simulink model "modelGreenHydrogenPlant"  (R2025a)
settings: Solver=ode1  StartTime=0.0  StopTime=exe.tsim  FixedStep=exe.tstep  RelTol=1e-3
undefined symbols (not defined in the file): Chosen_Strategy, DiscIntNeverNeededParam, ELY, ESS, exe, fb, Grid, grid, Ib2, Kc, kd, Ki_cc_cp, Ki_Inertia_Less, Kp_cc_cp, kp_GFo, Kp_Inertia_Less, PV, R, Rload, Sb, SCLR, t_ELY_on, Theta_Vvsc0, Time_Step, Va0, Vb0, Vb1, Vb2, Vc0, Vm0, VSC01_id0, Vvsc0, wb, Zb
libraries: spsSeriesRLCBranchLib x18, spsCurrentMeasurementLib x17, spsVoltageMeasurementLib x15, Control_Lib x13, spsRMSLib x8, simulink x8, spsabctodq0Lib x7, spsThreePhaseBreakerLib x5, spsPowerdq0InstantaneousLib x4, spsGroundLib x3, spsUniversalBridgeLib x3, spsControlledVoltageSourceLib x3
(part 2 of 3)

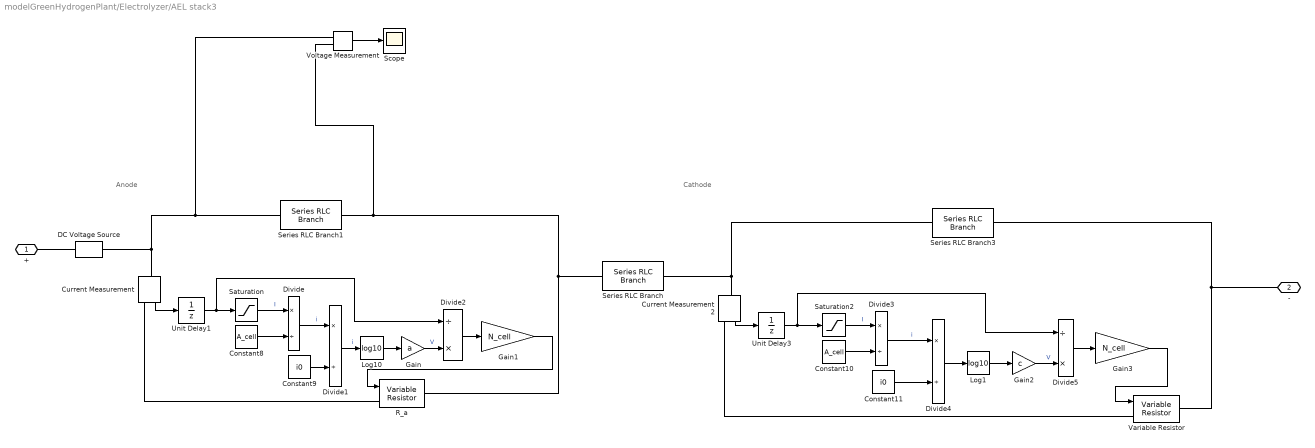
== system modelGreenHydrogenPlant/Electrolyzer/AEL stack3 ==
  note: Cathode
  note: Anode
  Constant10 : Constant  Value=A_cell
  Constant11 : Constant  Value=i0
  Constant8 : Constant  Value=A_cell
  Constant9 : Constant  Value=i0
  Current Measurement : spsCurrentMeasurementLib/Current Measurement  PhasorSimulation=off  OutputType=Complex  PSBequivalent=0
  Current Measurement2 : spsCurrentMeasurementLib/Current Measurement  PhasorSimulation=off  OutputType=Complex  PSBequivalent=0
  DC Voltage Source : spsDCVoltageSourceLib/DC Voltage Source  Amplitude=V_rev*N_cell  Measurements=None
  Divide{,1,3..4} (4 alike) : Product  Inputs=*/
  Divide2 : Product  Inputs=/*
  Divide5 : Product  Inputs=/*
  Gain : Gain  Gain=a
  Gain1 : Gain  Gain=N_cell
  Gain2 : Gain  Gain=c
  Gain3 : Gain  Gain=N_cell
  Log1 : Math  Operator=log10
  Log10 : Math  Operator=log10
  R_a : spsVariableResistorLib/Variable Resistor  Rabsmin=1e-3
      settings: LibrarySourceBlock=sps_lib/Passives/Variable Resistor
  Saturation : Saturate  UpperLimit=inf  LowerLimit=1e-3
  Saturation2 : Saturate  UpperLimit=inf  LowerLimit=1e-3
  Scope : Scope
      settings: ActiveDisplayYMinimum=40.73121  ActiveDisplayYMaximum=40.85796
  Series RLC Branch : spsSeriesRLCBranchLib/Series RLC Branch  LConnTagsString=__new0  RConnTagsString=__new0  BranchType=R  Resistance=R_cell_ohm/A_cell*N_cell  Inductance=1e-3  SetiL0=off  InitialCurrent=0  Capacitance=1e-6  Setx0=off  InitialVoltage=0  Measurements=None
  Series RLC Branch1 : spsSeriesRLCBranchLib/Series RLC Branch  LConnTagsString=__new0  RConnTagsString=__new0  BranchType=C  Resistance=1  Inductance=1e-3  SetiL0=off  InitialCurrent=0  Capacitance=Ca*A_cell *1e-3/N_cell  Setx0=on  InitialVoltage=V0_a_cell*N_cell  Measurements=None
  Series RLC Branch3 : spsSeriesRLCBranchLib/Series RLC Branch  LConnTagsString=__new0  RConnTagsString=__new0  BranchType=C  Resistance=1  Inductance=1e-3  SetiL0=off  InitialCurrent=0  Capacitance=Cc*A_cell *1e-3/N_cell  Setx0=on  InitialVoltage=V0_a_cell*N_cell  Measurements=None
  Unit Delay1 : UnitDelay  InitialCondition=I0_a  SampleTime=-1  HasFrameUpgradeWarning=on
  Unit Delay3 : UnitDelay  InitialCondition=I0_c  SampleTime=-1  HasFrameUpgradeWarning=on
  Variable Resistor : spsVariableResistorLib/Variable Resistor  Rabsmin=1e-3
      settings: LibrarySourceBlock=sps_lib/Passives/Variable Resistor
  Voltage Measurement : spsVoltageMeasurementLib/Voltage Measurement  PhasorSimulation=off  OutputType=Complex  PSBequivalent=0
  + : PMIOPort  Side=Left
  - : PMIOPort  Port=2  Side=Right
  wires:
  Saturation/1 -> Divide/1  "I"
  Constant8/1 -> Divide/2
  Gain/1 -> Divide2/2  "V"
  Gain1/1 -> R_a/1
  Divide2/1 -> Gain1/1
  Log10/1 -> Gain/1
  Current Measurement/1 -> Unit Delay1/1
  Current Measurement2/1 -> Unit Delay3/1
  Saturation2/1 -> Divide3/1  "I"
  Gain3/1 -> Variable Resistor/1
  Constant10/1 -> Divide3/2
  Divide5/1 -> Gain3/1
  Gain2/1 -> Divide5/2  "V"
  Divide4/1 -> Log1/1
  Log1/1 -> Gain2/1
  Constant11/1 -> Divide4/2
  Divide3/1 -> Divide4/1  "i"
  Divide/1 -> Divide1/1  "i"
  Constant9/1 -> Divide1/2
  Divide1/1 -> Log10/1  "i"
  Unit Delay1/1 -> Saturation/1, Divide2/1
  Unit Delay3/1 -> Divide5/1, Saturation2/1
  Voltage Measurement/1 -> Scope/1
  connections:
  R_a/RConn1 -- Voltage Measurement/LConn2 -- Series RLC Branch1/RConn1 -- Series RLC Branch/LConn1
  +/RConn1 -- DC Voltage Source/RConn1
  Current Measurement/RConn1 -- R_a/LConn1
  Series RLC Branch/RConn1 -- Current Measurement2/LConn1 -- Series RLC Branch3/LConn1
  Current Measurement2/RConn1 -- Variable Resistor/LConn1
  -/RConn1 -- Variable Resistor/RConn1 -- Series RLC Branch3/RConn1
  DC Voltage Source/LConn1 -- Current Measurement/LConn1 -- Voltage Measurement/LConn1 -- Series RLC Branch1/LConn1

== system modelGreenHydrogenPlant/Electrolyzer/Current Controller  ==
  Idref : Inport
  Iqref : Inport  Port=2
  Id : Inport  Port=3
  Iq : Inport  Port=4
  Vd : Inport  Port=5
  Vq : Inport  Port=6
  w : Inport  Port=7
  wt : Inport  Port=8
  Constant2 : Constant  Value=0
  Gain : Gain  Gain=ELY.CC.Kp
  Gain1 : Gain  Gain=ELY.CC.Ki
  Gain2 : Gain  Gain=ELY.CC.Kp
  Gain3 : Gain  Gain=ELY.CC.Ki
  Gain4 : Gain  Gain=ELY.CC.Lf
  Integrator : Integrator
  Integrator1 : Integrator
  Mux3 : Mux  Inputs=3
  Product : Product
  Product1 : Product
  Scope : Scope  NumInputPorts=2
      settings: ActiveDisplayYMinimum=-28.76857  ActiveDisplayYMaximum=18.72667
  Sum : Sum  Inputs=|+-
  Sum1 : Sum  Inputs=-+|
  Sum2 : Sum  Inputs=|++
  Sum3 : Sum  Inputs=|++
  Sum4 : Sum  Inputs=++-
  Sum5 : Sum  Inputs=+++
  dq0 to abc : spsdq0toabcLib/dq0 to abc  Alignment=90 degrees behind phase A axis
  Uref : Outport
  wires:
  Product/1 -> Sum4/3
  Product1/1 -> Sum5/1
  Idref/1 -> Sum/1
  Sum3/1 -> Sum5/2
  Integrator/1 -> Sum2/2
  Sum4/1 -> Mux3/1
  Integrator1/1 -> Sum3/2
  Constant2/1 -> Mux3/3
  Sum/1 -> Scope/1, Gain1/1, Gain/1
  Vd/1 -> Sum4/1
  Gain3/1 -> Integrator1/1
  Gain2/1 -> Sum3/1
  Gain/1 -> Sum2/1
  Gain4/1 -> Product/2, Product1/1
  Iq/1 -> Product/1, Sum1/1
  Id/1 -> Product1/2, Sum/2
  Sum2/1 -> Scope/2, Sum4/2
  Sum5/1 -> Mux3/2
  Sum1/1 -> Gain3/1, Gain2/1
  Gain1/1 -> Integrator/1
  Mux3/1 -> dq0 to abc/1
  dq0 to abc/1 -> Uref/1
  Iqref/1 -> Sum1/2
  w/1 -> Gain4/1
  wt/1 -> dq0 to abc/2
  Vq/1 -> Sum5/3

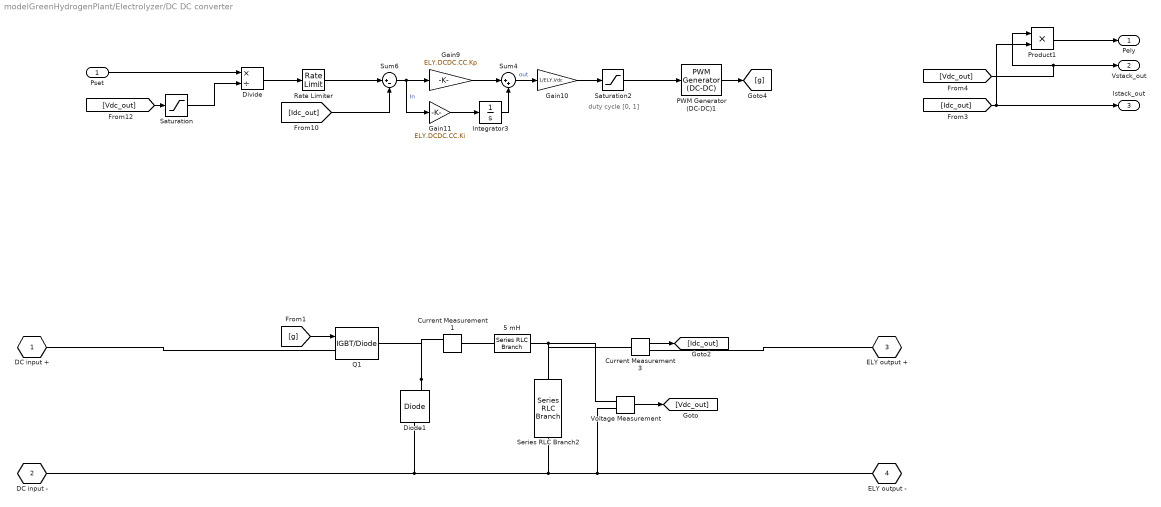
== system modelGreenHydrogenPlant/Electrolyzer/DC DC converter ==
  note: duty cycle [0, 1]
  Pset : Inport
  5 mH : spsSeriesRLCBranchLib/Series RLC Branch  LConnTagsString=__new0  RConnTagsString=__new0  BranchType=L  Resistance=ELY.DCDC.R_L  Inductance=ELY.DCDC.L  SetiL0=off  InitialCurrent=30  Capacitance=1.0  Setx0=off  InitialVoltage=0  Measurements=None
  Current Measurement1 : spsCurrentMeasurementLib/Current Measurement  PhasorSimulation=off  OutputType=Complex  PSBequivalent=0
  Current Measurement3 : spsCurrentMeasurementLib/Current Measurement  PhasorSimulation=off  OutputType=Complex  PSBequivalent=0
  Diode1 : spsDiodeLib/Diode  Ron=1e-3  Lon=0  Vf=0  IC=0  UseSnubber=off  Rs=inf  Cs=inf  Measurements=on
  Divide : Product  Inputs=*/
  Gain10 : Gain  Gain=1/ELY.Vdc
  Gain11 : Gain  Gain=ELY.DCDC.CC.Ki
  Gain9 : Gain  Gain=ELY.DCDC.CC.Kp
  Integrator3 : Integrator
  PWM Generator (DC-DC)1 : spsPWMGeneratorDCDCLib/PWM Generator (DC-DC)  Fsw=ELY.DCDC.fsw  Ts=0
  Product1 : Product
  Q1 : spsIGBTDiodeLib/IGBT//Diode  Ron=1e-3  Rs=1e5  Cs=inf  Measurements=off
  Rate Limiter : RateLimiter  RisingSlewLimit=ELY.DCDC.P.ramp.upperlimit  FallingSlewLimit=ELY.DCDC.P.ramp.lowerlimit  SampleTimeMode=inherited
  Saturation : Saturate  UpperLimit=inf  LowerLimit=95
  Saturation2 : Saturate  UpperLimit=1  LowerLimit=0
  Series RLC Branch2 : spsSeriesRLCBranchLib/Series RLC Branch  LConnTagsString=__new0  RConnTagsString=__new0  BranchType=C  Resistance=ELY.DCDC.R_C  Inductance=1e-3  SetiL0=off  InitialCurrent=0  Capacitance=20e-3+0*ELY.DCDC.C  Setx0=on  InitialVoltage=ELY.stack.Vstack  Measurements=None
  Sum4 : Sum  Inputs=|++
  Sum6 : Sum  Inputs=|+-
  Voltage Measurement : spsVoltageMeasurementLib/Voltage Measurement  PhasorSimulation=off  OutputType=Complex  PSBequivalent=0
  DC input + : PMIOPort  Tag=PMCPort  Side=Left
  DC input - : PMIOPort  Tag=PMCPort  Port=2  Side=Left
  ELY output + : PMIOPort  Tag=PMCPort  Port=3  Side=Right
  ELY output - : PMIOPort  Tag=PMCPort  Port=4  Side=Right
  Pely : Outport
  Vstack_out : Outport  Port=2
  Istack_out : Outport  Port=3
  wires:
  Current Measurement3/1 -> [Idc_out]
  [Idc_out] -> Istack_out/1, Product1/2
  [Vdc_out] -> Product1/1, Vstack_out/1
  Voltage Measurement/1 -> [Vdc_out]
  [g] -> Q1/1
  Gain10/1 -> Saturation2/1
  [Idc_out] -> Sum6/2
  Integrator3/1 -> Sum4/2
  Gain9/1 -> Sum4/1
  Sum6/1 -> Gain9/1, Gain11/1  "In"
  Gain11/1 -> Integrator3/1
  Saturation2/1 -> PWM Generator (DC-DC)1/1
  Sum4/1 -> Gain10/1  "out"
  PWM Generator (DC-DC)1/1 -> [g]
  Pset/1 -> Divide/1
  Divide/1 -> Rate Limiter/1
  Rate Limiter/1 -> Sum6/1
  Product1/1 -> Pely/1
  [Vdc_out] -> Saturation/1
  Saturation/1 -> Divide/2
  connections:
  Voltage Measurement/LConn2 -- ELY output -/RConn1 -- Diode1/LConn1 -- DC input -/RConn1 -- Series RLC Branch2/RConn1
  Diode1/RConn1 -- Current Measurement1/RConn1 -- Q1/RConn1
  DC input +/RConn1 -- Q1/LConn1
  Current Measurement1/LConn1 -- 5 mH/LConn1
  5 mH/RConn1 -- Voltage Measurement/LConn1 -- Current Measurement3/LConn1 -- Series RLC Branch2/LConn1
  Current Measurement3/RConn1 -- ELY output +/RConn1

== system modelGreenHydrogenPlant/Electrolyzer/PLL1 ==
  abc : Inport
  Add : Sum  Inputs=+++
  Add1 : Sum  Inputs=+++
  Constant : Constant  Value=2*pi*50
  Constant1 : Constant  Value=sqrt(2/3)*400
  Demux : Demux  Outputs=3
  Divide : Product  Inputs=*/
  Gain : Gain  Gain=ELY.PLL.kp
  Gain1 : Gain  Gain=ELY.PLL.ki
  Gain3 : Gain
  Gain7 : Gain  Gain=1/(2*pi)
  Integrator : Integrator
  Integrator1 : Integrator  InitialCondition=2*pi*50
  Sqrt : Sqrt
  Square : Math  Operator=square
  Square1 : Math  Operator=square
  Square2 : Math  Operator=square
  Terminator1 : Terminator
  abc to dq0 : spsabctodq0Lib/abc to dq0  Alignment=90 degrees behind phase A axis
  w : Outport
  Vd : Outport  Port=2
  Vq : Outport  Port=3
  wt : Outport  Port=4
  Vdq0 : Outport  Port=5
  Vamp : Outport  Port=6
  freq : Outport  Port=7
  Vamp_pu : Outport  Port=8
  wires:
  Integrator1/1 -> abc to dq0/2, wt/1
  Gain1/1 -> Integrator/1
  abc to dq0/1 -> Vdq0/1, Demux/1
  abc/1 -> abc to dq0/1
  Add/1 -> Gain7/1, w/1, Integrator1/1
  Demux/3 -> Square2/1, Terminator1/1
  Constant/1 -> Add/3
  Gain3/1 -> Gain/1, Gain1/1
  Square1/1 -> Add1/2
  Demux/2 -> Gain3/1, Square1/1, Vq/1
  Square/1 -> Add1/1
  Add1/1 -> Sqrt/1
  Demux/1 -> Vd/1, Square/1
  Sqrt/1 -> Divide/1, Vamp/1
  Gain7/1 -> freq/1  "freq"
  Constant1/1 -> Divide/2
  Divide/1 -> Vamp_pu/1
  Square2/1 -> Add1/3
  Gain/1 -> Add/1
  Integrator/1 -> Add/2

== system modelGreenHydrogenPlant/Electrolyzer/Subsystem ==
  Vd : Inport
  Vdc* : Inport  Port=2
  Vdc : Inport  Port=3
  Q* : Inport  Port=4
  Display : Display
  Divide : Product  Inputs=*/
  Divide1 : Product  Inputs=*/
  Gain : Gain  Gain=1e1%0.07%+ELY.DCV.Kp
  Gain1 : Gain  Gain=1%3.5%ELY.DCV.Ki*10
  Gain2 : Gain  Gain=2/3
  Gain3 : Gain  Gain=-2/3
  Gain4 : Gain  Gain=-1
  Integrator : Integrator
  Saturation : Saturate  UpperLimit=inf  LowerLimit=1e-8
  Saturation1 : Saturate  UpperLimit=inf  LowerLimit=1e-8
  Scope : Scope  NumInputPorts=2
      settings: ActiveDisplayYMinimum=-119.8458  ActiveDisplayYMaximum=13.4972
  Scope1 : Scope  NumInputPorts=2
      settings: ActiveDisplayYMinimum=665.50461  ActiveDisplayYMaximum=792.76508  DataLoggingVariableName=ScopeData2
  Sum : Sum  Inputs=|+-
  Sum1 : Sum  Inputs=|++
  idref : Outport
  iqref : Outport  Port=2
  wires:
  Vdc*/1 -> Scope1/1, Sum/1
  Vdc/1 -> Sum/2, Scope1/2
  Gain1/1 -> Integrator/1
  Integrator/1 -> Sum1/2
  Gain/1 -> Sum1/1
  Divide/1 -> Gain2/1
  Vd/1 -> Saturation1/1
  Saturation1/1 -> Saturation/1, Divide/2
  Gain3/1 -> Display/1, iqref/1
  Divide1/1 -> Gain3/1
  Saturation/1 -> Divide1/2
  Q*/1 -> Divide1/1
  Sum/1 -> Gain4/1
  Sum1/1 -> Scope/2, idref/1
  Gain4/1 -> Scope/1, Gain/1, Gain1/1

== system modelGreenHydrogenPlant/Electrolyzer/voltage conversion1 ==
  V_ll_abc : Inport
  Conversion to pu : Gain  Gain=1/PV.Vp
  Demux : Demux  Outputs=3
  Gain : Gain  Gain=-1/3
  Gain1 : Gain  Gain=1/3
  Gain2 : Gain  Gain=-1/3
  Mux : Mux  Inputs=3
  Sum : Sum  Inputs=|+-
  Sum1 : Sum  Inputs=|+-
  Sum2 : Sum  Inputs=|+-
  Vabc : Outport
  wires:
  V_ll_abc/1 -> Demux/1
  Demux/1 -> Sum1/2, Sum/2  "Vab"
  Demux/3 -> Sum/1, Sum2/2  "Vac"
  Sum/1 -> Gain/1
  Sum1/1 -> Gain1/1
  Sum2/1 -> Gain2/1
  Demux/2 -> Sum2/1, Sum1/1  "Vbc"
  Gain/1 -> Mux/1
  Gain1/1 -> Mux/2
  Gain2/1 -> Mux/3
  Mux/1 -> Vabc/1

== system modelGreenHydrogenPlant/Grid + SCLR/Grid  ==
  freq : Inport
  Vstep_pu : Inport  Port=2
  Add : Sum
  Add1 : Sum
  Add2 : Sum
  Constant3 : Constant  Value=0
  Constant4 : Constant  Value=-2*pi/3
  Constant5 : Constant  Value=+2*pi/3
  Constant6 : Constant  Value=grid.Vp
  Controlled Voltage Source : spsControlledVoltageSourceLib/Controlled Voltage Source  Initialize=off  Source_Type=AC  Amplitude=0  Phase=0  Frequency=0  Measurements=None
  Controlled Voltage Source1 : spsControlledVoltageSourceLib/Controlled Voltage Source  Initialize=off  Source_Type=AC  Amplitude=0  Phase=0  Frequency=0  Measurements=None
  Controlled Voltage Source2 : spsControlledVoltageSourceLib/Controlled Voltage Source  Initialize=off  Source_Type=AC  Amplitude=0  Phase=0  Frequency=0  Measurements=None
  Gain : Gain  Gain=2*pi
  Gain1 : Gain  Gain=2*pi
  Gain2 : Gain  Gain=2*pi
  Ground : spsGroundLib/Ground  LConnTagsString=a
  Integrator : Integrator  InitialCondition=2*pi*50
  Integrator1 : Integrator  InitialCondition=2*pi*50
  Integrator2 : Integrator  InitialCondition=2*pi*50
  Product{,1..3} (4 alike) : Product
  Trigonometric Function : Trigonometry  Operator=cos
  Trigonometric Function1 : Trigonometry  Operator=cos
  Trigonometric Function2 : Trigonometry  Operator=cos
  Ea : PMIOPort  Side=Right
  Eb : PMIOPort  Port=2  Side=Right
  Ec : PMIOPort  Port=3  Side=Right
  Theta : Outport
  wires:
  Constant3/1 -> Add/2
  Integrator/1 -> Add/1
  Gain/1 -> Integrator/1
  Constant5/1 -> Add2/2
  Integrator2/1 -> Add2/1
  Add/1 -> Theta/1, Trigonometric Function/1
  Product2/1 -> Controlled Voltage Source2/1
  Integrator1/1 -> Add1/1
  Add1/1 -> Trigonometric Function1/1
  Gain2/1 -> Integrator2/1
  freq/1 -> Gain/1, Gain1/1, Gain2/1
  Trigonometric Function1/1 -> Product1/1
  Constant4/1 -> Add1/2
  Trigonometric Function/1 -> Product/1
  Product1/1 -> Controlled Voltage Source1/1
  Gain1/1 -> Integrator1/1
  Product/1 -> Controlled Voltage Source/1
  Trigonometric Function2/1 -> Product2/1
  Add2/1 -> Trigonometric Function2/1
  Vstep_pu/1 -> Product3/1
  Constant6/1 -> Product3/2
  Product3/1 -> Product2/2, Product1/2, Product/2
  connections:
  Controlled Voltage Source/LConn1 -- Ground/LConn1 -- Controlled Voltage Source2/LConn1 -- Controlled Voltage Source1/LConn1
  Ec/RConn1 -- Controlled Voltage Source2/RConn1
  Eb/RConn1 -- Controlled Voltage Source1/RConn1
  Ea/RConn1 -- Controlled Voltage Source/RConn1

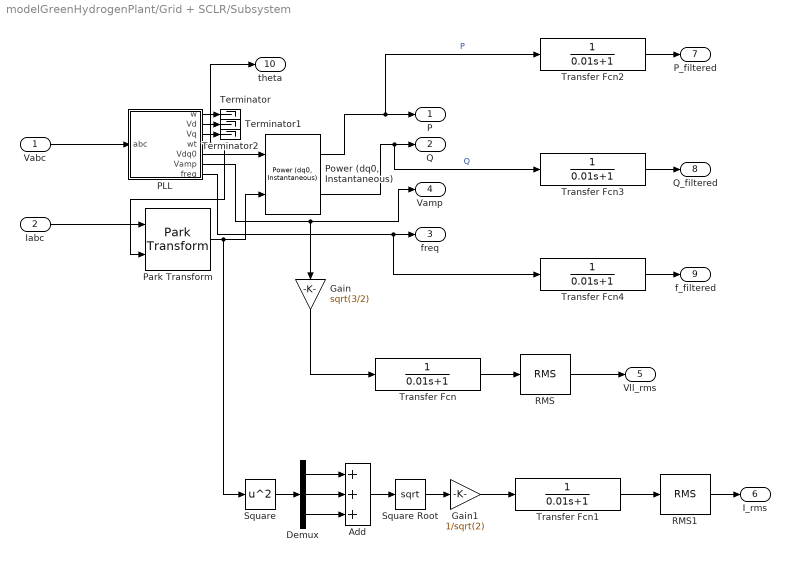
== system modelGreenHydrogenPlant/Grid + SCLR/Subsystem ==
  Vabc : Inport
  Iabc : Inport  Port=2
  Add : Sum  Inputs=+++
  Demux : Demux  Outputs=3
  Gain : Gain  Gain=sqrt(3/2)
  Gain1 : Gain  Gain=1/sqrt(2)
  PLL : Subsystem
  Park Transform : eeTransforms/Park Transform  AxisAlignment=Q-axis  PowerInvariant=off
      settings: LibrarySourceBlock=|
      | ee_sl_lib/Mathematical
      | Transforms/Park Transform
  "Power (dq0, Instantaneous)" : spsPowerdq0InstantaneousLib/Power (dq0, Instantaneous)
      settings: LibrarySourceBlock=|
      | sps_lib/Sensors and Measurements/Power
      | (dq0, Instantaneous)
  RMS : spsRMSLib/RMS  TrueRMS=on  Freq=50  RMSInit=400  Ts=0
  RMS1 : spsRMSLib/RMS  TrueRMS=on  Freq=50  RMSInit=0  Ts=0
  Square : Math  Operator=square
  Square Root : Sqrt
  Terminator : Terminator
  Terminator1 : Terminator
  Terminator2 : Terminator
  Transfer Fcn{,1..4} (5 alike) : TransferFcn  Denominator=[0.01 1]
  P : Outport
  Q : Outport  Port=2
  freq : Outport  Port=3
  Vamp : Outport  Port=4
  Vll_rms : Outport  Port=5
  I_rms : Outport  Port=6
  P_filtered : Outport  Port=7
  Q_filtered : Outport  Port=8
  f_filtered : Outport  Port=9
  theta : Outport  Port=10
  wires:
  PLL/1(w) -> Terminator/1
  Park Transform/1 -> Square/1, "Power (dq0, Instantaneous)"/2
  PLL/5(Vdq0) -> "Power (dq0, Instantaneous)"/1
  PLL/7(freq) -> Transfer Fcn4/1, freq/1
  PLL/4(wt) -> Park Transform/2, theta/1
  PLL/3(Vq) -> Terminator2/1
  Vabc/1 -> PLL/1(abc)
  "Power (dq0, Instantaneous)"/1 -> Transfer Fcn2/1, P/1  "P"
  PLL/2(Vd) -> Terminator1/1
  Iabc/1 -> Park Transform/1
  "Power (dq0, Instantaneous)"/2 -> Transfer Fcn3/1, Q/1  "Q"
  PLL/6(Vamp) -> Vamp/1, Gain/1
  Transfer Fcn/1 -> RMS/1
  RMS/1 -> Vll_rms/1
  Square/1 -> Demux/1
  Demux/3 -> Add/3
  Demux/2 -> Add/2
  Demux/1 -> Add/1
  Add/1 -> Square Root/1
  Transfer Fcn1/1 -> RMS1/1
  Square Root/1 -> Gain1/1
  Gain1/1 -> Transfer Fcn1/1
  Gain/1 -> Transfer Fcn/1
  RMS1/1 -> I_rms/1
  Transfer Fcn2/1 -> P_filtered/1
  Transfer Fcn3/1 -> Q_filtered/1
  Transfer Fcn4/1 -> f_filtered/1

== system modelGreenHydrogenPlant/PV plant/Active power control loop ==
  Pref_pu : Inport
  Vamp_pu_filtered : Inport  Port=2
  Voltage_dip : Inport  Port=3
  Add : Sum
  Avoiding divison by 0 : Saturate  UpperLimit=inf  LowerLimit=0.01
  Divide : Product  Inputs=*/
  Enabled Subsystem : Subsystem  TreatAsAtomicUnit=on
  NOT : Logic  Operator=NOT  IconShape=distinctive  AllPortsSameDT=off  OutDataTypeStr=boolean
  Pmin/Pmax : Saturate  UpperLimit=1  LowerLimit=0
  Product : Product
  Transfer Fcn : TransferFcn  Denominator=[PV.Tpord 1]
  dPmin/dPmax : RateLimiter  RisingSlewLimit=PV.dPmax  FallingSlewLimit=PV.dPmin  SampleTimeMode=inherited
  Ipcmd : Outport
  wires:
  Avoiding divison by 0/1 -> Divide/2
  Divide/1 -> Ipcmd/1
  Vamp_pu_filtered/1 -> Avoiding divison by 0/1
  Pref_pu/1 -> dPmin/dPmax/1
  dPmin/dPmax/1 -> Transfer Fcn/1
  Transfer Fcn/1 -> Pmin/Pmax/1
  Voltage_dip/1 -> Enabled Subsystem/Enable, NOT/1
  Add/1 -> Enabled Subsystem/1(In1), Divide/1
  Pmin/Pmax/1 -> Product/1
  Product/1 -> Add/2
  NOT/1 -> Product/2
  Enabled Subsystem/1(Out1) -> Add/1

== system modelGreenHydrogenPlant/PV plant/Current Controller  ==
  Idref_pu : Inport
  Iqref_pu : Inport  Port=2
  Id : Inport  Port=3
  Iq : Inport  Port=4
  Vd : Inport  Port=5
  Vq : Inport  Port=6
  w : Inport  Port=7
  wt : Inport  Port=8
  Constant2 : Constant  Value=0
  Gain : Gain  Gain=PV.CC.Kp
  Gain1 : Gain  Gain=PV.CC.Ki
  Gain2 : Gain  Gain=PV.CC.Kp
  Gain3 : Gain  Gain=PV.CC.Ki
  Gain4 : Gain  Gain=PV.Lc
  Integrator : Integrator
  Integrator1 : Integrator
  Mux3 : Mux  Inputs=3
  Product : Product
  Product1 : Product
  Sum : Sum  Inputs=|+-
  Sum1 : Sum  Inputs=-+|
  Sum2 : Sum  Inputs=|++
  Sum3 : Sum  Inputs=|++
  Sum4 : Sum  Inputs=++-
  Sum5 : Sum  Inputs=+++
  dq0 to abc : spsdq0toabcLib/dq0 to abc  Alignment=90 degrees behind phase A axis
  pu to ampere : Gain  Gain=2/3*50e3/(sqrt(2/3)*400)
  pu to ampere1 : Gain  Gain=2/3*50e3/(sqrt(2/3)*400)
  Uref : Outport
  wires:
  Vq/1 -> Sum5/3
  Product/1 -> Sum4/3
  Product1/1 -> Sum5/1
  Idref_pu/1 -> pu to ampere/1
  Sum3/1 -> Sum5/2
  Integrator/1 -> Sum2/2
  Sum4/1 -> Mux3/1
  Integrator1/1 -> Sum3/2
  Constant2/1 -> Mux3/3
  Vd/1 -> Sum4/1
  Gain3/1 -> Integrator1/1
  Gain2/1 -> Sum3/1
  Gain/1 -> Sum2/1
  Gain4/1 -> Product/2, Product1/1
  Iq/1 -> Product/1, Sum1/1
  Id/1 -> Product1/2, Sum/2
  Sum2/1 -> Sum4/2
  Sum5/1 -> Mux3/2
  Sum1/1 -> Gain3/1, Gain2/1
  Gain1/1 -> Integrator/1
  Mux3/1 -> dq0 to abc/1
  dq0 to abc/1 -> Uref/1
  w/1 -> Gain4/1
  wt/1 -> dq0 to abc/2
  Sum/1 -> Gain1/1, Gain/1
  pu to ampere/1 -> Sum/1
  Iqref_pu/1 -> pu to ampere1/1
  pu to ampere1/1 -> Sum1/2

== system modelGreenHydrogenPlant/PV plant/Current limit logic ==
  Vamp_pu_filtered : Inport
  Iqcmd : Inport  Port=2
  Active V-I : Lookup_n-D  NumberOfTableDimensions=1  BreakpointsForDimension1=[0; 0.9]  Table=[ 0; 1]  InternalRulePriority=Speed  RndMeth=Simplest
  Add : Sum  Inputs=-+
  Constant : Constant  Value=PV.Imax
  Constant1 : Constant  Value=PV.Imax
  Constant2 : Constant  Value=0
  Gain : Gain  Gain=-1
  Min : MinMax  Inputs=2
  Min1 : MinMax  Inputs=2
  Reactive V-I : Lookup_n-D  NumberOfTableDimensions=1  BreakpointsForDimension1=[ 0; 1]  Table=[ 0; 0.9]  InternalRulePriority=Speed  RndMeth=Simplest
  Square : Math  Operator=square
  Square Root : Sqrt
  Square1 : Math  Operator=square
  Ipmax : Outport
  Ipmin : Outport  Port=2
  Iqmax : Outport  Port=3
  Iqmin : Outport  Port=4
  wires:
  Vamp_pu_filtered/1 -> Active V-I/1, Reactive V-I/1
  Constant/1 -> Square/1
  Iqcmd/1 -> Square1/1
  Square1/1 -> Add/1
  Square/1 -> Add/2
  Add/1 -> Square Root/1
  Constant1/1 -> Min/2
  Reactive V-I/1 -> Min/1
  Min/1 -> Iqmax/1, Gain/1
  Gain/1 -> Iqmin/1
  Square Root/1 -> Min1/1
  Active V-I/1 -> Min1/2
  Min1/1 -> Ipmax/1
  Constant2/1 -> Ipmin/1

== system modelGreenHydrogenPlant/PV plant/PLL ==
  abc : Inport
  Add : Sum  Inputs=+++
  Add1 : Sum
  Constant : Constant  Value=2*pi*50
  Constant1 : Constant  Value=sqrt(2/3)*400
  Demux : Demux  Outputs=3
  Divide : Product  Inputs=*/
  Gain : Gain  Gain=PV.PLL.kp
  Gain1 : Gain  Gain=PV.PLL.ki
  Gain3 : Gain
  Gain7 : Gain  Gain=1/(2*pi)
  Integrator : Integrator
  Integrator1 : Integrator  InitialCondition=2*pi*50
  Sqrt : Sqrt
  Square : Math  Operator=square
  Square1 : Math  Operator=square
  Terminator1 : Terminator
  abc to dq0 : spsabctodq0Lib/abc to dq0  Alignment=90 degrees behind phase A axis
  w : Outport
  Vd : Outport  Port=2
  Vq : Outport  Port=3
  wt : Outport  Port=4
  Vdq0 : Outport  Port=5
  Vamp : Outport  Port=6
  freq : Outport  Port=7
  Vamp_pu : Outport  Port=8
  wires:
  Integrator1/1 -> abc to dq0/2, wt/1
  Gain/1 -> Add/1
  Integrator/1 -> Add/2
  Gain1/1 -> Integrator/1
  abc to dq0/1 -> Vdq0/1, Demux/1
  abc/1 -> abc to dq0/1
  Add/1 -> Gain7/1, w/1, Integrator1/1
  Demux/3 -> Terminator1/1
  Constant/1 -> Add/3
  Gain3/1 -> Gain/1, Gain1/1
  Square1/1 -> Add1/2
  Demux/2 -> Gain3/1, Square1/1, Vq/1
  Square/1 -> Add1/1
  Add1/1 -> Sqrt/1
  Demux/1 -> Square/1, Vd/1
  Sqrt/1 -> Divide/1, Vamp/1
  Gain7/1 -> freq/1  "freq"
  Constant1/1 -> Divide/2
  Divide/1 -> Vamp_pu/1

== system modelGreenHydrogenPlant/PV plant/Reactive power control loop ==
  Pe_pu : Inport
  Vamp_pu_filtered : Inport  Port=2
  Add : Sum
  Avoiding divison by 0 : Saturate  UpperLimit=inf  LowerLimit=0.01
  Divide : Product  Inputs=*/
  Product : Product
  Transfer Fcn : TransferFcn  Denominator=[PV.Tiq 1]
  Transfer Fcn1 : TransferFcn  Denominator=[PV.Tp 1]
  Voltage dip controller : Subsystem
  tan(theta) : Constant  Value=tan(0)
  Iqcmd : Outport
  Voltage_dip : Outport  Port=2
  wires:
  Avoiding divison by 0/1 -> Divide/2
  Pe_pu/1 -> Transfer Fcn1/1
  Divide/1 -> Transfer Fcn/1
  Transfer Fcn1/1 -> Product/2
  tan(theta)/1 -> Product/1
  Product/1 -> Divide/1
  Add/1 -> Iqcmd/1
  Vamp_pu_filtered/1 -> Voltage dip controller/1(Vamp_pu_filtered), Avoiding divison by 0/1
  Voltage dip controller/1(Iqref) -> Add/2
  Transfer Fcn/1 -> Add/1
  Voltage dip controller/2(Voltage_dip) -> Voltage_dip/1

== system modelGreenHydrogenPlant/PV plant/voltage conversion ==
  V_ll_abc : Inport
  Conversion to pu : Gain  Gain=1/PV.Vp
  Demux : Demux  Outputs=3
  Gain : Gain  Gain=-1/3
  Gain1 : Gain  Gain=1/3
  Gain2 : Gain  Gain=-1/3
  Mux : Mux  Inputs=3
  Sum : Sum  Inputs=|+-
  Sum1 : Sum  Inputs=|+-
  Sum2 : Sum  Inputs=|+-
  Vabc : Outport
  wires:
  V_ll_abc/1 -> Demux/1
  Demux/1 -> Sum1/2, Sum/2  "Vab"
  Demux/3 -> Sum/1, Sum2/2  "Vac"
  Sum/1 -> Gain/1
  Sum1/1 -> Gain1/1
  Sum2/1 -> Gain2/1
  Demux/2 -> Sum2/1, Sum1/1  "Vbc"
  Gain/1 -> Mux/1
  Gain1/1 -> Mux/2
  Gain2/1 -> Mux/3
  Mux/1 -> Vabc/1

== system modelGreenHydrogenPlant/Supercapacitor/GFM_VC_newwith_Pvirt IDEAL_VSC ==
  note: Control part
  note: Measurements and normalization
  note: Power part
  note: Common Inputs
  note: do not modify this part if you use the update loaflow script
  dE_set (pu) : Inport
  dP_set (pu) : Inport  Port=2
  1/Ib2 : Gain  Gain=1/Vb2
  1/Ib3 : Gain  Gain=1/Ib2
  Add : Sum
  Add1 : Sum
  Bridge_Model : Subsystem
  Bus01 : spsThreePhaseVIMeasurementLib/Three-Phase V-I Measurement  VoltageMeasurement=phase-to-ground  SetLabelV=off  LabelV=Vabc  Vpu=off  VpuLL=off  CurrentMeasurement=yes  SetLabelI=off  LabelI=Iabc  Ipu=off  Pbase=100e6  Vbase=500e3  OutputType=Complex  PhasorSimulation=off  PSBequivalent=0
  Control loops2 : Subsystem
  DC_Link : Source_Lib/DC_Link  Udc=Udcn  Pb=Pn  H_DC=H_DC
      settings: SourceProductName=Voltage Source
  Delay : Delay  Commented=through  DelayLength=1
  Delay1 : Delay  Commented=through  DelayLength=1
  Display : Display
  Display1 : Display
  Output_Transformer : spsThreePhaseTransformerTwoWindingsLib/Three-Phase Transformer (Two Windings)  Winding1Connection=Yg  Winding2Connection=Yg  CoreType=Three single-phase transformers  SetSaturation=off  Hysteresis=off  DataFile='hysteresis'  SetInitialFlux=off  Measurements=None  UNITS=pu  NominalPower=[Sn , fb]  Winding1=[Un1 , Rt_pu/2 , Lt_pu/2]  Winding2=[Un2 , Rt_pu/2 , Lt_pu/2]  Rm=Rm_pu  Lm=Lm_pu  L0=0.5  Saturation=[ 0,0 ; 0.0024,1.2 ; 1.0,1.52 ]  InitialFluxes=[ 0.8 , -0.8 , 0.7 ]  BreakLoop=off  DiscreteSolver=Trapezoidal iterative  DataType=off  TransfoNumber=1
  Pinit : Constant  Value=0
  Source_For_LF : spsThreePhaseSourceLib/Three-Phase Source  Commented=on  InternalConnection=Yg  VoltagePhases=off  Voltage=(400000)*1  PhaseAngle=2.5991  Voltage_phases=[25e3 25e3 25e3]/sqrt(3)  PhaseAngles_phases=[0 -120 +120]  Frequency=fb  NonIdealSource=off  SpecifyImpedance=off  Resistance=0  Inductance=0  ShortCircuitLevel=100e6  BaseVoltage=Un  XRratio=7  BusType=PV  Pref=P0*Sb  Qref=Q0*Sb  Prefabc=[10e3, 10e3, 10e3]  Qrefabc=[0, 0, 0]  Qmin=-inf  Qmax=inf
  Transport Delay : TransportDelay  DelayTime=Output_Delay  InitialOutput=[Va0 Vb0 Vc0]
  Vvsc_init : Constant  Value=Vvsc0
  mp3 : Gain  Gain=Vb1
  A : PMIOPort  Side=Right
  B : PMIOPort  Port=2  Side=Right
  C : PMIOPort  Port=3  Side=Right
  + : PMIOPort  Port=4  Side=Left
  - : PMIOPort  Port=5  Side=Left
  m : Outport  VectorParamsAs1DForOutWhenUnconnected=off
  wires:
  Bus01/2 -> [ig_meas]
  dE_set (pu)/1 -> Add1/1
  Bus01/1 -> [vg_meas]
  Vvsc_init/1 -> Add1/2
  Pinit/1 -> Add/2
  dP_set (pu)/1 -> Add/1
  Transport Delay/1 -> Bridge_Model/1(Uref)
  Add1/1 -> Display1/1, Control loops2/1(E_set)
  Control loops2/1(vm_abc_ref_pu) -> mp3/1
  1/Ib2/1 -> Control loops2/3(vg_abc_pu)  "vg_pu"
  1/Ib3/1 -> Control loops2/4(ig_abc_pu)  "ig_pu"
  mp3/1 -> Transport Delay/1
  Control loops2/2(m) -> m/1  "Control"
  Add/1 -> Display/1, Control loops2/2(P_set)
  Delay/1 -> 1/Ib2/1
  [vg_meas] -> Delay/1
  [ig_meas] -> Delay1/1
  Delay1/1 -> 1/Ib3/1
  connections:
  DC_Link/RConn3 -- -/RConn1 -- Bridge_Model/LConn2
  DC_Link/RConn1 -- +/RConn1 -- Bridge_Model/LConn1
  Bus01/RConn3 -- C/RConn1 -- Source_For_LF/RConn3
  Bus01/RConn1 -- A/RConn1 -- Source_For_LF/RConn1
  Bridge_Model/RConn3 -- Output_Transformer/LConn3
  Bridge_Model/RConn2 -- Output_Transformer/LConn2
  Bridge_Model/RConn1 -- Output_Transformer/LConn1
  Bus01/RConn2 -- B/RConn1 -- Source_For_LF/RConn2
  Output_Transformer/RConn3 -- Bus01/LConn3
  Output_Transformer/RConn2 -- Bus01/LConn2
  Output_Transformer/RConn1 -- Bus01/LConn1

== system modelGreenHydrogenPlant/Supercapacitor/PLL1 ==
  abc : Inport
  Add : Sum  Inputs=+++
  Add1 : Sum  Inputs=+++
  Constant : Constant  Value=2*pi*50
  Constant1 : Constant  Value=sqrt(2/3)*400
  Demux : Demux  Outputs=3
  Divide : Product  Inputs=*/
  Gain : Gain  Gain=ELY.PLL.kp
  Gain1 : Gain  Gain=ELY.PLL.ki
  Gain3 : Gain
  Gain7 : Gain  Gain=1/(2*pi)
  Integrator : Integrator
  Integrator1 : Integrator  InitialCondition=2*pi*50
  Sqrt : Sqrt
  Square : Math  Operator=square
  Square1 : Math  Operator=square
  Square2 : Math  Operator=square
  Terminator1 : Terminator
  abc to dq0 : spsabctodq0Lib/abc to dq0  Alignment=90 degrees behind phase A axis
  w : Outport
  Vd : Outport  Port=2
  Vq : Outport  Port=3
  wt : Outport  Port=4
  Vdq0 : Outport  Port=5
  Vamp : Outport  Port=6
  freq : Outport  Port=7
  Vamp_pu : Outport  Port=8
  wires:
  Integrator1/1 -> abc to dq0/2, wt/1
  Gain/1 -> Add/1
  Integrator/1 -> Add/2
  Gain1/1 -> Integrator/1
  abc to dq0/1 -> Vdq0/1, Demux/1
  abc/1 -> abc to dq0/1
  Add/1 -> Gain7/1, w/1, Integrator1/1
  Demux/3 -> Square2/1, Terminator1/1
  Constant/1 -> Add/3
  Gain3/1 -> Gain/1, Gain1/1
  Square1/1 -> Add1/2
  Demux/2 -> Gain3/1, Square1/1, Vq/1
  Square/1 -> Add1/1
  Add1/1 -> Sqrt/1
  Demux/1 -> Vd/1, Square/1
  Sqrt/1 -> Divide/1, Vamp/1
  Gain7/1 -> freq/1  "freq"
  Constant1/1 -> Divide/2
  Divide/1 -> Vamp_pu/1
  Square2/1 -> Add1/3

== system modelGreenHydrogenPlant/Supercapacitor/voltage conversion1 ==
  V_ll_abc : Inport
  Conversion to pu : Gain  Gain=1/PV.Vp
  Demux : Demux  Outputs=3
  Gain : Gain  Gain=-1/3
  Gain1 : Gain  Gain=1/3
  Gain2 : Gain  Gain=-1/3
  Mux : Mux  Inputs=3
  Sum : Sum  Inputs=|+-
  Sum1 : Sum  Inputs=|+-
  Sum2 : Sum  Inputs=|+-
  Vabc : Outport
  wires:
  V_ll_abc/1 -> Demux/1
  Demux/1 -> Sum1/2, Sum/2  "Vab"
  Demux/3 -> Sum/1, Sum2/2  "Vac"
  Sum/1 -> Gain/1
  Sum1/1 -> Gain1/1
  Sum2/1 -> Gain2/1
  Demux/2 -> Sum2/1, Sum1/1  "Vbc"
  Gain/1 -> Mux/1
  Gain1/1 -> Mux/2
  Gain2/1 -> Mux/3
  Mux/1 -> Vabc/1

== system modelGreenHydrogenPlant/Grid + SCLR/Subsystem/PLL ==
  abc : Inport
  Add : Sum  Inputs=+++
  Add1 : Sum  Inputs=+++
  Constant : Constant  Value=2*pi*50
  Demux : Demux  Outputs=3
  Gain : Gain  Gain=PV.PLL.kp
  Gain1 : Gain  Gain=PV.PLL.ki
  Gain2 : Gain  Gain=1/(2*pi)
  Gain3 : Gain  Gain=-1
  Integrator : Integrator
  Integrator1 : Integrator  InitialCondition=2*pi*50
  Square : Math  Operator=square
  Square Root : Sqrt
  Square1 : Math  Operator=square
  Square2 : Math  Operator=square
  Terminator1 : Terminator
  abc to dq0 : spsabctodq0Lib/abc to dq0  Alignment=90 degrees behind phase A axis
  w : Outport
  Vd : Outport  Port=2
  Vq : Outport  Port=3
  wt : Outport  Port=4
  Vdq0 : Outport  Port=5
  Vamp : Outport  Port=6
  freq : Outport  Port=7
  wires:
  Integrator1/1 -> abc to dq0/2, wt/1
  Gain/1 -> Add/1
  Demux/2 -> Gain3/1, Square1/1, Vq/1
  Integrator/1 -> Add/2
  Gain1/1 -> Integrator/1
  abc to dq0/1 -> Vdq0/1, Demux/1
  abc/1 -> abc to dq0/1
  Add/1 -> Gain2/1, w/1, Integrator1/1
  Demux/1 -> Square/1, Vd/1
  Demux/3 -> Square2/1, Terminator1/1
  Constant/1 -> Add/3
  Gain3/1 -> Gain/1, Gain1/1
  Square/1 -> Add1/1
  Square1/1 -> Add1/2
  Square2/1 -> Add1/3
  Add1/1 -> Square Root/1
  Square Root/1 -> Vamp/1
  Gain2/1 -> freq/1

== system modelGreenHydrogenPlant/PV plant/Active power control loop/Enabled Subsystem ==
  In1 : Inport
  Enable : EnablePort
  Out1 : Outport
  wires:
  In1/1 -> Out1/1

== system modelGreenHydrogenPlant/PV plant/Reactive power control loop/Voltage dip controller ==
  Vamp_pu_filtered : Inport
  Constant : Constant  Value=PV.Vref0
  Constant1 : Constant  Value=0
  Constant2 : Constant
  Constant3 : Constant  Value=0
  Dead Zone1 : DeadZone  LowerValue=PV.dbd1  UpperValue=PV.dbd2
  Gain : Gain  Gain=PV.Kqv
  If : If  IfExpression=u1<0.9|u1>1.1
  If Action Subsystem : Subsystem  TreatAsAtomicUnit=on
  If Action Subsystem1 : Subsystem  TreatAsAtomicUnit=on
  Merge : Merge
  Saturation : Saturate  UpperLimit=PV.Iqh1  LowerLimit=PV.Iql1
  Scope1 : Scope  NumInputPorts=2
      settings: ActiveDisplayYMinimum=-0.05169  ActiveDisplayYMaximum=0.46519  DataLoggingVariableName=ScopeData10
  Sum : Sum  Inputs=|-+
  Switch : Switch  Criteria=u2 ~= 0  SaturateOnIntegerOverflow=off  InputSameDT=off
  Iqref : Outport
  Voltage_dip : Outport  Port=2
  wires:
  Vamp_pu_filtered/1 -> Sum/1, If/1
  Constant/1 -> Sum/2
  Gain/1 -> Scope1/1, Saturation/1
  If/2 -> If Action Subsystem/Action
  Constant1/1 -> If Action Subsystem/1(In1)
  If/1 -> If Action Subsystem1/Action
  Constant2/1 -> If Action Subsystem1/1(In1)
  If Action Subsystem1/1(Out1) -> Merge/1
  If Action Subsystem/1(Out1) -> Merge/2
  Merge/1 -> Switch/2, Voltage_dip/1
  Switch/1 -> Iqref/1
  Saturation/1 -> Switch/1
  Constant3/1 -> Switch/3
  Dead Zone1/1 -> Gain/1
  Sum/1 -> Dead Zone1/1

== system modelGreenHydrogenPlant/Supercapacitor/GFM_VC_newwith_Pvirt IDEAL_VSC/Bridge_Model ==
  Uref : Inport
  NOT1 : Logic  Operator=NOT  IconShape=distinctive  AllPortsSameDT=off  OutDataTypeStr=boolean
  Saturation : Saturate  UpperLimit=1  LowerLimit=-1
  Scope : Scope  NumInputPorts=2
      settings: ActiveDisplayYMinimum=-1.11775  ActiveDisplayYMaximum=1.11082
  Step : Step  Time=Output_Delay  SampleTime=0
  Three-Phase Breaker1 : spsThreePhaseBreakerLib/Three-Phase Breaker  InitialState=closed  SwitchA=on  SwitchB=on  SwitchC=on  SwitchTimes="[4/60  10/60]"  External=on  BreakerResistance=1e-5*Zb  SnubberResistance=1e6  SnubberCapacitance=inf  Measurements=None
  Three-Phase Breaker2 : spsThreePhaseBreakerLib/Three-Phase Breaker  InitialState=open  SwitchA=on  SwitchB=on  SwitchC=on  SwitchTimes="[4/60  10/60]"  External=on  BreakerResistance=1e-5*Zb  SnubberResistance=1e6  SnubberCapacitance=inf  Measurements=None
  Three-Phase Source : spsThreePhaseSourceLib/Three-Phase Source  InternalConnection=Yg  VoltagePhases=off  Voltage=Vm0*Un1  PhaseAngle=Theta_Vm0  Voltage_phases=[25e3 25e3 25e3]/sqrt(3)  PhaseAngles_phases=[0 -120 +120]  Frequency=fb  NonIdealSource=off  SpecifyImpedance=off  Resistance=0  Inductance=0  ShortCircuitLevel=100e6  BaseVoltage=VSC01_Un1  XRratio=7  BusType=swing  Pref=0.3  Qref=0  Prefabc=[10e3, 10e3, 10e3]  Qrefabc=[0, 0, 0]  Qmin=-Inf  Qmax=Inf
  Universal Bridge : spsUniversalBridgeLib/Universal Bridge  Arms=3  SnubberResistance=1e5  SnubberCapacitance=inf  Device=Average-model based VSC  Ron=1e-3  Lon=0  ForwardVoltages="[  0  0  ]"  ForwardVoltage=0  GTOparameters=[ 10e-6 , 20e-6 ]  IGBTparameters=[ 1e-6 , 2e-6 ]  Measurements=None  Measurements_2=None  converterType=Rectifier
  mp3 : Gain  Gain=2/Udcn
  PhA : PMIOPort  Side=Right
  PhB : PMIOPort  Port=2  Side=Right
  PhC : PMIOPort  Port=3  Side=Right
  Vdc+ : PMIOPort  Port=4  Side=Left
  Vdc- : PMIOPort  Port=5  Side=Left
  wires:
  Uref/1 -> Scope/1, mp3/1
  mp3/1 -> Scope/2, Saturation/1
  Step/1 -> NOT1/1, Three-Phase Breaker2/1
  NOT1/1 -> Three-Phase Breaker1/1
  Saturation/1 -> Universal Bridge/1
  connections:
  Universal Bridge/RConn2 -- Vdc-/RConn1
  Universal Bridge/RConn1 -- Vdc+/RConn1
  Three-Phase Source/RConn3 -- Three-Phase Breaker1/RConn3
  Three-Phase Source/RConn2 -- Three-Phase Breaker1/RConn2
  Three-Phase Source/RConn1 -- Three-Phase Breaker1/RConn1
  Three-Phase Breaker2/RConn3 -- Universal Bridge/LConn3
  Three-Phase Breaker2/RConn2 -- Universal Bridge/LConn2
  Three-Phase Breaker2/RConn1 -- Universal Bridge/LConn1
  PhC/RConn1 -- Three-Phase Breaker1/LConn3 -- Three-Phase Breaker2/LConn3
  PhB/RConn1 -- Three-Phase Breaker1/LConn2 -- Three-Phase Breaker2/LConn2
  PhA/RConn1 -- Three-Phase Breaker1/LConn1 -- Three-Phase Breaker2/LConn1

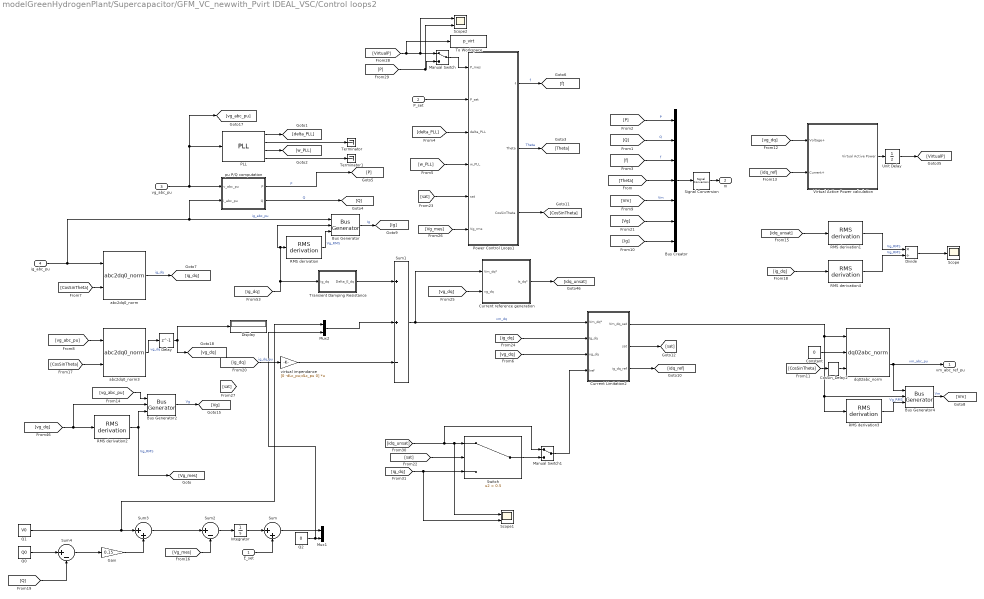
== system modelGreenHydrogenPlant/Supercapacitor/GFM_VC_newwith_Pvirt IDEAL_VSC/Control loops2 ==
  E_set : Inport
  P_set : Inport  Port=2
  vg_abc_pu : Inport  Port=3
  ig_abc_pu : Inport  Port=4
  " pu P/Q computation" : Subsystem  DialogController=POWERSYS.PowerSysDialog
  Bus Creator : BusCreator  Inputs=7
  Bus Generator : Control_Lib/Bus Generator  Gpu=Ib2
      settings: SourceProductName=Control
  Bus Generator2 : Control_Lib/Bus Generator  Gpu=Vb2
      settings: SourceProductName=Control
  Bus Generator4 : Control_Lib/Bus Generator  Gpu=Vb1
      settings: SourceProductName=Control
  Constant : Constant  Value=0
  CosSin_Delay2 : Control_Lib/CosSin_Delay  dTheta=wb*(Output_Delay)
      settings: SourceProductName=Control
  Current Limitation2 : Subsystem
  Current reference generation : Subsystem  mask{Tau_fCC=0.01, Lt=Lt_pu}
      mask prompts: Tau_fCC "Tau_f"; Lt "Model impedance"
  Delay : Delay  DelayLength=1  InitialCondition=[1 0]
  Display : Display
  Divide : Product  Inputs=*/
  Gain : Gain  Gain=0.15
  Integrator : Integrator
  Manual Switch : ManualSwitch
  Manual Switch1 : ManualSwitch
  Mux1 : Mux  Inputs=2
  Mux2 : Mux  Inputs=2
  PLL : Control_Lib/PLL  fb=fb  wn_PLL=wn_PLL  zeta_PLL=zeta_PLL  Theta0=Theta0
      settings: SourceProductName=Control
  Power Control Loops1 : Subsystem  AncestorBlock=Control_Lib/Power Control Loops  mask{Theta0_VSC=Theta_Vvsc0}
      mask prompts: Theta0_VSC "Initial VSC angle"
      mask DialogControl DescGroupVar Prompt: Parameters
  Q0 : Constant  Value=Q0
  Q1 : Constant  Value=V0
  Q2 : Constant  Value=0
  RMS derivation{,1..4} (5 alike) : Control_Lib/RMS derivation  SystemSampleTime=-1  VariantActivationTime=update diagram  EmptyChoice=off  PassThrough=off  PassThroughVariantControl=(default)  EmptyChoiceVariantControl=(default)  AllowFlexibleInterface=on  Latency=0  AutoFrameSizeCalculation=off
      settings: SourceProductName=Control
  Scope : Scope
      settings: ActiveDisplayYMinimum=-0.33796  ActiveDisplayYMaximum=12.16108
  Scope1 : Scope  NumInputPorts=2
      settings: ActiveDisplayYMinimum=-1.4846  ActiveDisplayYMaximum=2.46905  DataLoggingVariableName=ScopeData2
  Scope2 : Scope  NumInputPorts=2
      settings: ActiveDisplayYMinimum=-0.24195  ActiveDisplayYMaximum=2.73076
  Signal Conversion : SignalConversion  OverrideOpt=off
  Sum : Sum  Inputs=|++
  Sum1 : Sum  Inputs=++-
  Sum2 : Sum  Inputs=|+-
  Sum3 : Sum  Inputs=|++
  Sum4 : Sum  Inputs=|+-
  Switch : Switch  Criteria=u2 > Threshold  Threshold=0.5  SaturateOnIntegerOverflow=off  InputSameDT=off
  Terminator : Terminator
  Terminator1 : Terminator
  To Workspace : ToWorkspace  VariableName=p_virt  SaveFormat=Timeseries  SampleTime=-1
  Transient Damping Resistance : Subsystem
  Unit Delay : UnitDelay  InitialCondition=P0  SampleTime=-1  HasFrameUpgradeWarning=on
  Virtual Active Power calculation : Subsystem
  abc2dq0_norm : Control_Lib/abc2dq0_norm  referenceAxisMode=Reference axis at 90 degrees behind phase_a  baseUpdateGain=1/sqrt(3)
      settings: SourceProductName=Control
  abc2dq0_norm3 : Control_Lib/abc2dq0_norm  referenceAxisMode=Reference axis at 90 degrees behind phase_a  baseUpdateGain=1/sqrt(3)
      settings: SourceProductName=Control
  dq02abc_norm : Control_Lib/dq02abc_norm  referenceAxisMode=Reference axis at 90 degrees behind phase_a  baseUpdateGain=sqrt(3)
      settings: SourceProductName=Control
  virtual impendance : Gain  Gain=[0 -dLc_pu;dLc_pu 0]  Multiplication=Matrix(K*u)
  vm_abc_ref_pu : Outport  PortDimensions=3  VectorParamsAs1DForOutWhenUnconnected=off
  m : Outport  Port=2  VectorParamsAs1DForOutWhenUnconnected=off
  wires:
  [Ig] -> Bus Creator/7
  [Vg] -> Bus Creator/6
  RMS derivation3/1 -> Bus Generator4/3  "Vg_RMS"
  Bus Generator4/1 -> [Vm]  "Vm"
  [CosSinTheta] -> abc2dq0_norm3/2
  [vg_abc_pu] -> abc2dq0_norm3/1
  abc2dq0_norm3/2 -> Delay/1  "vg_dq"
  [vg_abc_pu] -> Bus Generator2/1
  RMS derivation2/1 -> Bus Generator2/3, [Vg_mes]  "Vg_RMS"
  Bus Generator2/1 -> [Vg]  "Vg"
  RMS derivation/1 -> Bus Generator/3  "Vg_RMS"
  CosSin_Delay2/1 -> dq02abc_norm/3
  PLL/4 -> Terminator1/1
  PLL/2 -> Terminator/1
  Constant/1 -> dq02abc_norm/2
  Power Control Loops1/3(CosSinTheta) -> [CosSinTheta]
  PLL/3 -> [w_PLL]
  PLL/1 -> [delta_PLL]
  dq02abc_norm/2 -> vm_abc_ref_pu/1, Bus Generator4/1  "vm_abc_pu"
  vg_abc_pu/1 -> [vg_abc_pu], PLL/1, " pu P/Q computation"/1(v_abc_pu)
  Bus Generator/1 -> [Ig]  "Ig"
  Bus Creator/1 -> Signal Conversion/1
  [Vm] -> Bus Creator/5  "Vm"
  Transient Damping Resistance/1("Delta_E_dq ") -> Sum1/1
  [CosSinTheta] -> abc2dq0_norm/2
  Power Control Loops1/2(Theta) -> [Theta]  "Theta"
  abc2dq0_norm/2 -> [ig_dq]  "ig_dq"
  " pu P/Q computation"/1(P) -> [P]  "P"
  Power Control Loops1/1(f) -> [f]  "f"
  [w_PLL] -> Power Control Loops1/4(w_PLL)
  P_set/1 -> Power Control Loops1/2(P_set)
  [delta_PLL] -> Power Control Loops1/3(delta_PLL)
  " pu P/Q computation"/2(Q) -> [Q]  "Q"
  [f] -> Bus Creator/3  "f"
  [Q] -> Bus Creator/2  "Q"
  [P] -> Bus Creator/1  "P"
  Signal Conversion/1 -> m/1
  [idq_ref] -> Virtual Active Power calculation/2(Current+)
  Virtual Active Power calculation/1(Virtual Active Power) -> Unit Delay/1
  [vg_dq] -> Virtual Active Power calculation/1(Voltage+)
  Unit Delay/1 -> [VirtualP]
  [vg_dq] -> Current reference generation/2(vg_dq)
  Current reference generation/1(Is_dq*) -> [idq_unsat]
  Manual Switch/1 -> Power Control Loops1/1(P_mes)
  [VirtualP] -> To Workspace/1, Scope2/1, Manual Switch/1
  [P] -> Scope2/2, Manual Switch/2
  ig_abc_pu/1 -> abc2dq0_norm/1, Bus Generator/1, " pu P/Q computation"/2(i_abc_pu)  "ig_abc_pu"
  [vg_dq] -> Bus Generator2/2, RMS derivation2/1
  [ig_dq] -> Transient Damping Resistance/1(ig_dq), Bus Generator/2, RMS derivation/1
  [Theta] -> Bus Creator/4
  [CosSinTheta] -> CosSin_Delay2/1
  [ig_dq] -> Current Limitation2/2(Ig_dq)
  [vg_dq] -> Current Limitation2/3(vg_dq)
  Sum1/1 -> Current Limitation2/1(Vm_dq*), Current reference generation/1(Vm_dq*)  "vm_dq"
  Current Limitation2/3(ig_dq_ref) -> [idq_ref]
  [idq_unsat] -> RMS derivation1/1
  [ig_dq] -> RMS derivation4/1
  RMS derivation1/1 -> Divide/1  "Vg_RMS"
  RMS derivation4/1 -> Divide/2  "Vg_RMS"
  Divide/1 -> Scope/1
  Current Limitation2/1(Vm_dq_sat) -> RMS derivation3/1, Bus Generator4/2, dq02abc_norm/1
  Sum4/1 -> Gain/1
  Gain/1 -> Sum3/2
  [Q] -> Sum4/2
  Integrator/1 -> Sum/1
  Q2/1 -> Mux2/2, Mux1/2
  Q1/1 -> Mux2/1, Sum3/1
  Q0/1 -> Sum4/1
  Sum/1 -> Mux1/1
  [Vg_mes] -> Sum2/2
  Sum2/1 -> Integrator/1
  E_set/1 -> Sum/2
  Sum3/1 -> Sum2/1
  [ig_dq] -> virtual impendance/1  "ig_dq_pu"
  Current Limitation2/2(sat) -> [sat]
  [sat] -> Switch/2
  [ig_dq] -> Scope1/2, Switch/3
  [sat] -> Power Control Loops1/5(sat)
  [Vg_mes] -> Power Control Loops1/6(Vg_rms)
  Switch/1 -> Manual Switch1/2
  [idq_unsat] -> Manual Switch1/1, Scope1/1, Switch/1
  Manual Switch1/1 -> Current Limitation2/4(Iref)
  Mux2/1 -> Sum1/2
  virtual impendance/1 -> Sum1/3
  Delay/1 -> [vg_dq], Display/1

== system modelGreenHydrogenPlant/PV plant/Reactive power control loop/Voltage dip controller/If Action Subsystem ==
  In1 : Inport
  Action Port : ActionPort  ActionPortLabel=else
  Out1 : Outport
  wires:
  In1/1 -> Out1/1

== system modelGreenHydrogenPlant/PV plant/Reactive power control loop/Voltage dip controller/If Action Subsystem1 ==
  In1 : Inport
  Action Port : ActionPort  ActionPortLabel=if(u1<0.9|u1>1.1)
  Out1 : Outport
  wires:
  In1/1 -> Out1/1

== system modelGreenHydrogenPlant/Supercapacitor/GFM_VC_newwith_Pvirt IDEAL_VSC/Control loops2/ pu P//Q computation ==
  v_abc_pu : Inport  PortDimensions=3
  i_abc_pu : Inport  Port=2  PortDimensions=3
  Demux : Demux  Outputs=3
      settings: DisplayOption=none
  Mux : Mux  Inputs=3
  Product1 : Product  InputSameDT=on  SaturateOnIntegerOverflow=on  OutDataTypeStr=Inherit: Same as first input
  Product3 : Product  InputSameDT=on  SaturateOnIntegerOverflow=on  OutDataTypeStr=Inherit: Same as first input
  Sum : Sum  Inputs=+-  InputSameDT=on  SaturateOnIntegerOverflow=on  OutDataTypeStr=Inherit: Same as first input
  Sum1 : Sum  Inputs=1  InputSameDT=on  SaturateOnIntegerOverflow=on  OutDataTypeStr=Inherit: Same as first input
  Sum4 : Sum  Inputs=1  InputSameDT=on  SaturateOnIntegerOverflow=on  OutDataTypeStr=Inherit: Same as first input
  Sum5 : Sum  Inputs=+-  InputSameDT=on  SaturateOnIntegerOverflow=on  OutDataTypeStr=Inherit: Same as first input
  Sum6 : Sum  Inputs=+-  InputSameDT=on  SaturateOnIntegerOverflow=on  OutDataTypeStr=Inherit: Same as first input
  pu->V : Gain  Gain=1/sqrt(3)  SaturateOnIntegerOverflow=on  OutDataTypeStr=Inherit: Same as input  ParamDataTypeStr=Inherit: Same as input
  pu->V1 : Gain  Gain=1/3  SaturateOnIntegerOverflow=on  OutDataTypeStr=Inherit: Same as input  ParamDataTypeStr=Inherit: Same as input
  pu->V2 : Gain  Gain=1/3  SaturateOnIntegerOverflow=on  OutDataTypeStr=Inherit: Same as input  ParamDataTypeStr=Inherit: Same as input
  P : Outport  VectorParamsAs1DForOutWhenUnconnected=off
  Q : Outport  Port=2  VectorParamsAs1DForOutWhenUnconnected=off
  wires:
  pu->V2/1 -> Q/1
  pu->V1/1 -> P/1
  Sum1/1 -> pu->V/1
  Product3/1 -> Sum1/1
  Product1/1 -> Sum4/1
  v_abc_pu/1 -> Product1/1, Demux/1
  i_abc_pu/1 -> Product1/2, Product3/2
  Sum4/1 -> pu->V1/1
  Demux/1 -> Sum/1, Sum6/2
  Demux/2 -> Sum/2, Sum5/1
  Demux/3 -> Sum5/2, Sum6/1
  Sum/1 -> Mux/3
  Sum5/1 -> Mux/1
  Sum6/1 -> Mux/2
  Mux/1 -> Product3/1
  pu->V/1 -> pu->V2/1  "Q"

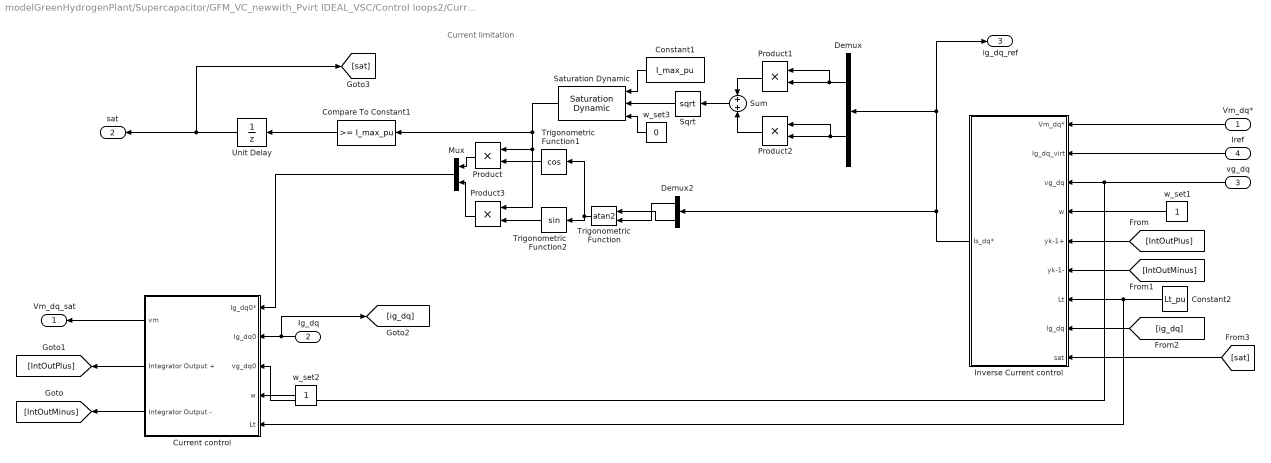
== system modelGreenHydrogenPlant/Supercapacitor/GFM_VC_newwith_Pvirt IDEAL_VSC/Control loops2/Current Limitation2 ==
  note: Current limitation
  Vm_dq* : Inport
  Ig_dq : Inport  Port=2
  vg_dq : Inport  Port=3
  Iref : Inport  Port=4
  Compare To Constant1 : simulink/Logic and Bit Operations/Compare To Constant  relop=>=  const=I_max_pu  OutDataTypeStr=boolean
  Constant1 : Constant  Value=I_max_pu
  Constant2 : Constant  Value=Lt_pu
  Current control : Subsystem
  Demux : Demux  Outputs=2
  Demux2 : Demux  Outputs=2
  Inverse Current control : Subsystem
  Mux : Mux  Inputs=2
  Product{,1..3} (4 alike) : Product
  Saturation Dynamic : simulink/Discontinuities/Saturation Dynamic  OutMin=[]  OutMax=[]  OutDataTypeStr=Inherit: Same as second input  OutDataType=fixdt(1, 16)  OutScaling=2^-10  DoSatur=off
  Sqrt : Sqrt
  Sum : Sum
  Trigonometric Function : Trigonometry  Operator=atan2  NumberOfIterations=5  OutputSignalType=real
  Trigonometric Function1 : Trigonometry  Operator=cos
  Trigonometric Function2 : Trigonometry
  Unit Delay : UnitDelay  SampleTime=-1  HasFrameUpgradeWarning=on
  w_set1 : Constant
  w_set2 : Constant
  w_set3 : Constant  Value=0
  Vm_dq_sat : Outport  VectorParamsAs1DForOutWhenUnconnected=off
  sat : Outport  Port=2
  ig_dq_ref : Outport  Port=3
  wires:
  w_set3/1 -> Saturation Dynamic/3
  Product/1 -> Mux/1
  Demux/1 -> Product1/1, Product1/2
  Demux/2 -> Product2/1, Product2/2
  Trigonometric Function2/1 -> Product3/2
  Product2/1 -> Sum/2
  Trigonometric Function1/1 -> Product/2
  Demux2/1 -> Trigonometric Function/2
  Trigonometric Function/1 -> Trigonometric Function2/1, Trigonometric Function1/1
  Product1/1 -> Sum/1
  Sqrt/1 -> Saturation Dynamic/2
  Demux2/2 -> Trigonometric Function/1
  Sum/1 -> Sqrt/1
  Product3/1 -> Mux/2
  Ig_dq/1 -> [ig_dq], Current control/2(Ig_dq0)
  w_set1/1 -> Inverse Current control/4(w)
  w_set2/1 -> Current control/4(w)
  Vm_dq*/1 -> Inverse Current control/1(Vm_dq*)
  Current control/1(vm) -> Vm_dq_sat/1
  Mux/1 -> Current control/1(Ig_dq0*)
  vg_dq/1 -> Current control/3(vg_dq0), Inverse Current control/3(vg_dq)
  Current control/3(Integrator Output -) -> [IntOutMinus]
  [IntOutMinus] -> Inverse Current control/6(yk-1-)
  Current control/2(Integrator Output +) -> [IntOutPlus]
  [IntOutPlus] -> Inverse Current control/5(yk-1+)
  Constant1/1 -> Saturation Dynamic/1
  Saturation Dynamic/1 -> Compare To Constant1/1, Product/1, Product3/1
  Compare To Constant1/1 -> Unit Delay/1
  Constant2/1 -> Current control/5(Lt), Inverse Current control/7(Lt)
  Iref/1 -> Inverse Current control/2(Ig_dq_virt)
  Inverse Current control/1(Is_dq*) -> Demux2/1, ig_dq_ref/1, Demux/1
  [ig_dq] -> Inverse Current control/8(Ig_dq)
  [sat] -> Inverse Current control/9(sat)
  Unit Delay/1 -> [sat], sat/1

== system modelGreenHydrogenPlant/Supercapacitor/GFM_VC_newwith_Pvirt IDEAL_VSC/Control loops2/Current reference generation ==
  Vm_dq* : Inport
  vg_dq : Inport  Port=2
  Add2 : Sum  Inputs=+++
  Add3 : Sum  Inputs=+-
  Constant : Constant  Value=10e-3
  Constant2 : Constant  Value=V0
  Constant5 : Constant  Value=Lt_pu
  Constant6 : Constant
  Constant7 : Constant  Value=13e-2
  Demux : Demux  Outputs=2
  Demux2 : Demux  Outputs=2
  Divide1 : Product  Inputs=*/
  Gain : Gain  Gain=-1
  Gain2 : Gain  Gain=inv([Rt_pu -Lt_pu;+Lt_pu Rt_pu])  Multiplication=Matrix(K*u)
  Manual Switch : ManualSwitch  CurrentSetting=0
  Manual Switch1 : ManualSwitch
  Mux : Mux  Inputs=2
  Mux1 : Mux  Inputs=2
  Product1 : Product
  Product2 : Product
  Product3 : Product
  RMS2 : Subsystem
  Saturation1 : Saturate  UpperLimit=0  LowerLimit=-0.14
  Scope4 : Scope
      settings: ActiveDisplayYMinimum=-0.09981  ActiveDisplayYMaximum=1.13534  DataLoggingVariableName=ScopeData2
  Scope5 : Scope
      settings: ActiveDisplayYMinimum=-0.43314  ActiveDisplayYMaximum=0.04813  DataLoggingVariableName=ScopeData3
  Subsystem : Subsystem
  Subsystem1 : Subsystem
  Sum4 : Sum  Inputs=|+-
  Unit Delay1 : UnitDelay  SampleTime=-1  HasFrameUpgradeWarning=on
  Is_dq* : Outport  InitialOutput=0  VectorParamsAs1DForOutWhenUnconnected=off
  wires:
  Unit Delay1/1 -> Manual Switch1/1
  Manual Switch1/1 -> Add2/1
  Vm_dq*/1 -> Sum4/1
  Demux2/2 -> Subsystem1/2(In1)
  Demux2/1 -> Subsystem/1(In1)
  Subsystem/1(Out1) -> Mux1/1
  Subsystem1/1(Out1) -> Mux1/2
  vg_dq/1 -> RMS2/1(Is_dq*), Demux2/1
  Sum4/1 -> Gain2/1, Demux/1
  Mux1/1 -> Sum4/2
  Constant/1 -> Subsystem1/1(tau_f), Subsystem/2(tau_f)
  Demux/2 -> Product1/1
  Product1/1 -> Mux/1
  Product2/1 -> Gain/1
  Demux/1 -> Product2/2
  Manual Switch/1 -> Is_dq*/1
  Gain2/1 -> Manual Switch/1
  Mux/1 -> Manual Switch/2
  Constant5/1 -> Add2/2
  Constant6/1 -> Divide1/1
  Divide1/1 -> Product2/1, Product1/2
  Gain/1 -> Mux/2
  Add2/1 -> Divide1/2
  Product3/1 -> Saturation1/1
  Constant2/1 -> Add3/2
  Constant7/1 -> Product3/1
  Add3/1 -> Product3/2
  RMS2/1(Out1) -> Add3/1, Scope4/1
  Saturation1/1 -> Unit Delay1/1, Scope5/1
